simulink model "L1E4_DC_Motor_Speed_Model"  (R2019b)
settings: Solver=VariableStepAuto  StartTime=0.0  StopTime=5  RelTol=1e-3
model workspace (MAT data in the model file):
  k = Simulink.Parameter
  k.Value = 5.7
  k.DataType = 'auto'
  k.Dimensions = [1 1]
  m = Simulink.Parameter
  m.DataType = 'auto'
  m.Dimensions = [0 0]
  wn = Simulink.Parameter
  wn.Value = 1
  wn.DataType = 'auto'
  wn.Dimensions = [1 1]
  zeta = Simulink.Parameter
  zeta.Value = 5
  zeta.DataType = 'auto'
  zeta.Dimensions = [1 1]
undefined symbols (not defined in the file or in its folder): b, J, K, L, R
settings Model: Creator=Callum  LastModifiedBy=Callum
settings DataIOCC: ReturnWorkspaceOutputs=off

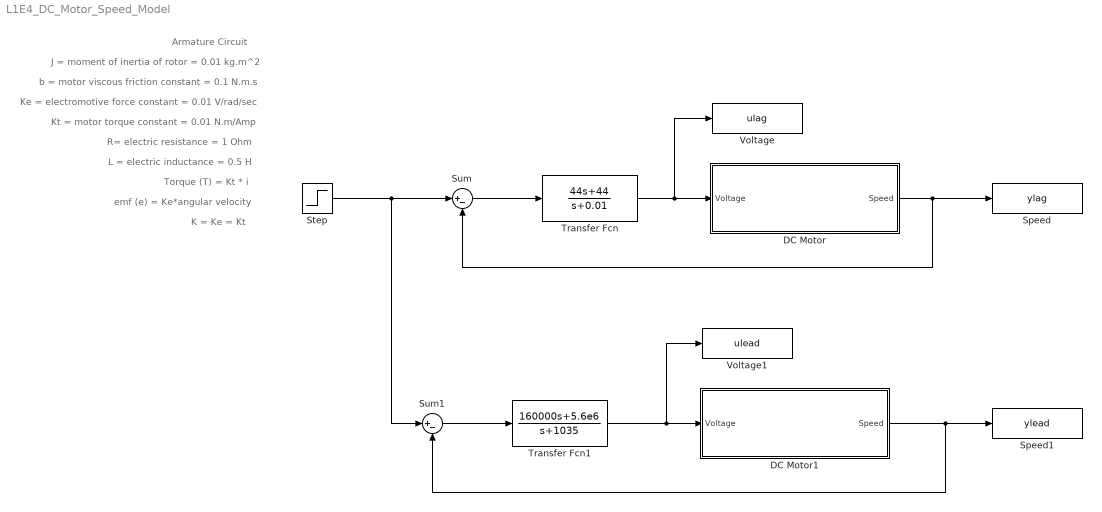
== system L1E4_DC_Motor_Speed_Model ==
  note: Armature Circuit
  note: K = Ke = Kt
  note: emf (e) = Ke*angular velocity
  note: Torque (T) = Kt * i
  note: L = electric inductance = 0.5 H
  note: R= electric resistance = 1 Ohm
  note: Kt = motor torque constant = 0.01 N.m/Amp
  note: Ke = electromotive force constant = 0.01 V/rad/sec
  note: b = motor viscous friction constant = 0.1 N.m.s
  note: J = moment of inertia of rotor = 0.01 kg.m^2
  DC Motor : Subsystem
  DC Motor1 : Subsystem
  Speed : ToWorkspace  VariableName=ylag  SampleTime=-1
  Speed1 : ToWorkspace  VariableName=ylead  SaveFormat=Timeseries  SampleTime=-1
  Step : Step  SampleTime=0
  Sum : Sum  Inputs=|+-
  Sum1 : Sum  Inputs=|+-
  Transfer Fcn : TransferFcn  Numerator=[44 44]  Denominator=[1 0.01]
  Transfer Fcn1 : TransferFcn  Numerator=[160000 5.6e6]  Denominator=[1 1035]
  Voltage : ToWorkspace  VariableName=ulag  SampleTime=-1
  Voltage1 : ToWorkspace  VariableName=ulead  SampleTime=-1
  wires:
  DC Motor/1(Speed) -> Speed/1, Sum/2
  Transfer Fcn/1 -> Voltage/1, DC Motor/1(Voltage)
  Sum/1 -> Transfer Fcn/1
  Sum1/1 -> Transfer Fcn1/1
  Transfer Fcn1/1 -> Voltage1/1, DC Motor1/1(Voltage)
  Step/1 -> Sum1/1, Sum/1
  DC Motor1/1(Speed) -> Speed1/1, Sum1/2

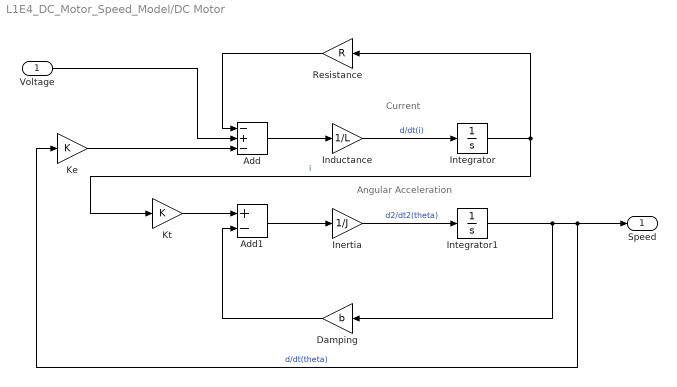
== system L1E4_DC_Motor_Speed_Model/DC Motor ==
  note: Angular Acceleration
  note: Current
  Voltage : Inport
  Add : Sum  Inputs=-+-
  Add1 : Sum  Inputs=+-
  Damping : Gain  Gain=b
  Inductance : Gain  Gain=1/L
  Inertia : Gain  Gain=1/J
  Integrator : Integrator
  Integrator1 : Integrator
  Ke : Gain  Gain=K
  Kt : Gain  Gain=K
  Resistance : Gain  Gain=R
  Speed : Outport
  wires:
  Inertia/1 -> Integrator1/1  "d2/dt2(theta)"
  Add1/1 -> Inertia/1
  Integrator/1 -> Kt/1, Resistance/1  "i"
  Inductance/1 -> Integrator/1  "d/dt(i)"
  Ke/1 -> Add/3
  Kt/1 -> Add1/1
  Integrator1/1 -> Speed/1, Ke/1, Damping/1  "d/dt(theta)"
  Damping/1 -> Add1/2
  Resistance/1 -> Add/1
  Add/1 -> Inductance/1
  Voltage/1 -> Add/2

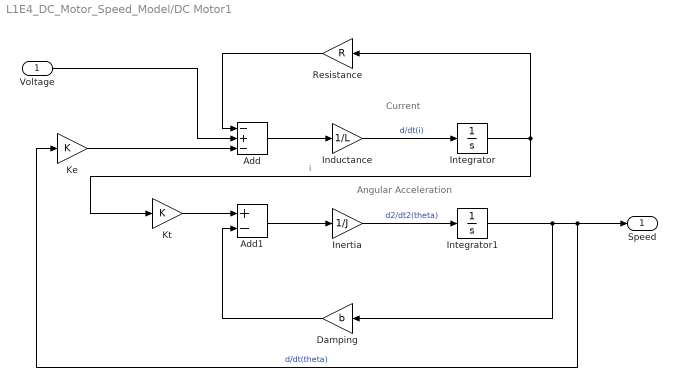
== system L1E4_DC_Motor_Speed_Model/DC Motor1 ==
  note: Angular Acceleration
  note: Current
  Voltage : Inport
  Add : Sum  Inputs=-+-
  Add1 : Sum  Inputs=+-
  Damping : Gain  Gain=b
  Inductance : Gain  Gain=1/L
  Inertia : Gain  Gain=1/J
  Integrator : Integrator
  Integrator1 : Integrator
  Ke : Gain  Gain=K
  Kt : Gain  Gain=K
  Resistance : Gain  Gain=R
  Speed : Outport
  wires:
  Inertia/1 -> Integrator1/1  "d2/dt2(theta)"
  Add1/1 -> Inertia/1
  Integrator/1 -> Kt/1, Resistance/1  "i"
  Inductance/1 -> Integrator/1  "d/dt(i)"
  Ke/1 -> Add/3
  Kt/1 -> Add1/1
  Integrator1/1 -> Speed/1, Ke/1, Damping/1  "d/dt(theta)"
  Damping/1 -> Add1/2
  Resistance/1 -> Add/1
  Add/1 -> Inductance/1
  Voltage/1 -> Add/2
